simulink model "vrs_inflow_testbench"  (R2024a)
settings: Solver=ode45  StartTime=0.0  StopTime=40  MaxStep=0.05  RelTol=1e-3
InitFcn:
  | init_vrs_model
values from neighbouring files (symbols this model uses):
  P_vrs = vrs_params()    [init_vrs_model.m]
  vi0 = hover.v_i_qs    [init_vrs_model.m]
settings Model: Creator=26534  LastModifiedBy=26534

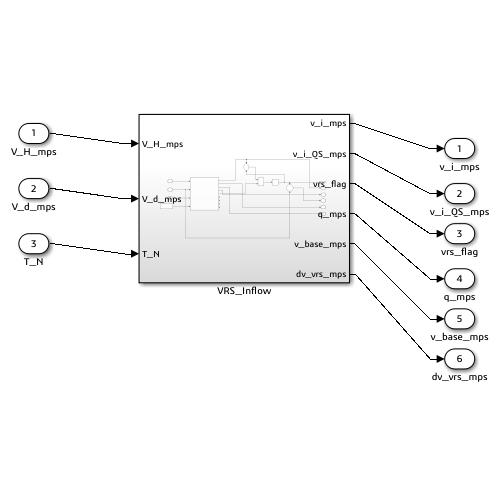
[thumbnail: Simulink's stored preview of the top-level diagram]
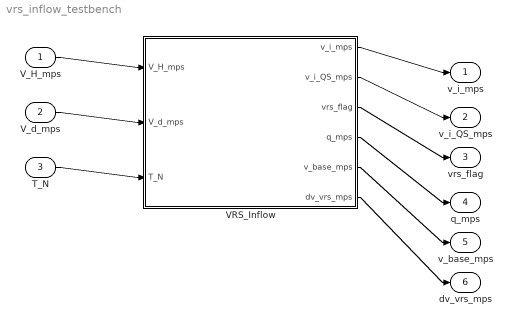
== system vrs_inflow_testbench ==
  V_H_mps : Inport
  V_d_mps : Inport  Port=2
  T_N : Inport  Port=3
  VRS_Inflow : Subsystem
  v_i_mps : Outport
  v_i_QS_mps : Outport  Port=2
  vrs_flag : Outport  Port=3
  q_mps : Outport  Port=4
  v_base_mps : Outport  Port=5
  dv_vrs_mps : Outport  Port=6
  wires:
  V_H_mps/1 -> VRS_Inflow/1(V_H_mps)
  V_d_mps/1 -> VRS_Inflow/2(V_d_mps)
  T_N/1 -> VRS_Inflow/3(T_N)
  VRS_Inflow/1(v_i_mps) -> v_i_mps/1
  VRS_Inflow/2(v_i_QS_mps) -> v_i_QS_mps/1
  VRS_Inflow/3(vrs_flag) -> vrs_flag/1
  VRS_Inflow/4(q_mps) -> q_mps/1
  VRS_Inflow/5(v_base_mps) -> v_base_mps/1
  VRS_Inflow/6(dv_vrs_mps) -> dv_vrs_mps/1

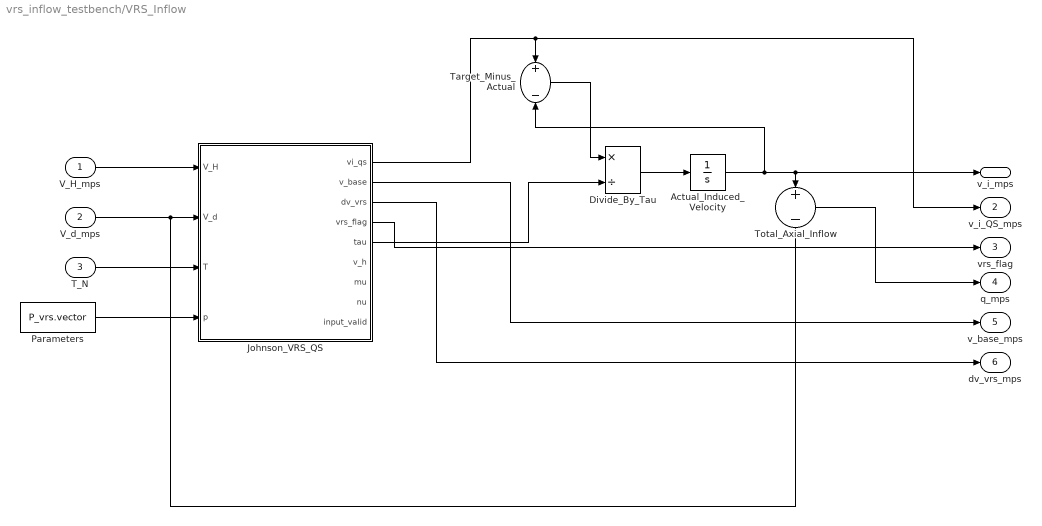
== system vrs_inflow_testbench/VRS_Inflow ==
  V_H_mps : Inport
  V_d_mps : Inport  Port=2
  T_N : Inport  Port=3
  Actual_Induced_Velocity : Integrator  InitialCondition=vi0
  Divide_By_Tau : Product  Inputs=*/
  Johnson_VRS_QS : MATLAB Function  TreatAsAtomicUnit=on
  Parameters : Constant  Value=P_vrs.vector
  Target_Minus_Actual : Sum  Inputs=+-
  Total_Axial_Inflow : Sum  Inputs=+-
  v_i_mps : Outport
  v_i_QS_mps : Outport  Port=2
  vrs_flag : Outport  Port=3
  q_mps : Outport  Port=4
  v_base_mps : Outport  Port=5
  dv_vrs_mps : Outport  Port=6
  wires:
  V_H_mps/1 -> Johnson_VRS_QS/1(V_H)
  V_d_mps/1 -> Johnson_VRS_QS/2(V_d), Total_Axial_Inflow/2
  T_N/1 -> Johnson_VRS_QS/3(T)
  Parameters/1 -> Johnson_VRS_QS/4(p)
  Johnson_VRS_QS/1(vi_qs) -> Target_Minus_Actual/1, v_i_QS_mps/1
  Actual_Induced_Velocity/1 -> Target_Minus_Actual/2, v_i_mps/1, Total_Axial_Inflow/1
  Target_Minus_Actual/1 -> Divide_By_Tau/1
  Johnson_VRS_QS/5(tau) -> Divide_By_Tau/2
  Divide_By_Tau/1 -> Actual_Induced_Velocity/1
  Johnson_VRS_QS/4(vrs_flag) -> vrs_flag/1
  Total_Axial_Inflow/1 -> q_mps/1
  Johnson_VRS_QS/2(v_base) -> v_base_mps/1
  Johnson_VRS_QS/3(dv_vrs) -> dv_vrs_mps/1

== matlab function vrs_inflow_testbench/VRS_Inflow/Johnson_VRS_QS ==
  data: V_H input; vi_qs output; V_d input; T input; p input; v_base output; dv_vrs output; vrs_flag output; tau output; v_h output; mu output; nu output; input_valid output
function [vi_qs,v_base,dv_vrs,vrs_flag,tau,v_h,mu,nu,input_valid] = fcn(V_H,V_d,T,p)
%#codegen
[vi_qs,v_base,dv_vrs,vrs_flag,tau,v_h,mu,nu,input_valid] = ...
    vrs_johnson_qs_numeric(V_H,V_d,T,p);
end
